simulink model "rect_v_RRC"  (R2014b)
settings: Solver=VariableStepDiscrete  StartTime=0.0  StopTime=5000/fs  RelTol=1e-3
PreLoadFcn:
  | %%%%%%%%%%%%%%%%%%%%%%%%%%%%%%%%%%%%%%%%%%%%%%%%%%%%%%%%%%%%%%%%%%%%%%%%%%%
  | % check to see if Simulink library folder is missing from the MATLAB path %
  | %%%%%%%%%%%%%%%%%%%%%%%%%%%%%%%%%%%%%%%%%%%%%%%%%%%%%%%%%%%%%%%%%%%%%%%%%%%
  | if isempty(strfind(path, 'rtlsdr_book_library'))
  | 
  |     % create error window
  |     fig_error = figure(...
  |         'Name', 'Error: RTL-SDR Book Library',...
  |         'Toolbar','none',...
  |         'MenuBar','none',...
  |         'NumberTitle','off',...
  |         'Resize','off',...
  |         'WindowStyle','modal');
  |     fig_error.Position(3) = 600;
  |     fig_error.Position(4) = 150;
  |     fig_axes = axes(...
  |         'Parent',fig_error,...
  |         'Position',[0,0,1,1],...
  |         'visible','off');
  |     % error message
  |     t_title = text(.05,.8,...
  |         'MISSING DIRECTORIES',...
  |         'FontSize',11.5);
  |     t_body = text(.075,.6,...
  |         [{'Simulink cannot find the  \it{<root>}\rm / \it{rtlsdr\_book\_library}\rm  folder in the \it{MATLAB Path}\rm.'},...
  |         {'Please set the MATLAB path following the instructions given in Exercise 2.4.'}],...
  |         'FontSize',10.5);
  |     % buttons
  |     btn_path = uicontrol(...
  |         'Parent',fig_error,...
  |         'String','Set Path Now',...
  |         'FontSize',10,...
  |         'Callback', 'pathtool; close(fig_error);',...
  |         'Position', [fig_error.Position(3)/2-210, 30, 200, 30]);
  |     btn_abort = uicontrol(...
  |         'Parent',fig_error,...
  |         'String','No thanks',...
  |         'FontSize',10,...
  |         'Callback', 'close(fig_error); abort=1;',...
  |         'Position', [fig_error.Position(3)/2+10, 30, 200, 30]);
  | 
  |     % pause to allow user to interact with error box
  |     uiwait(fig_error);
  | 
  |     % abort simulation
  |     try
  |         if abort==1
  |             set_param(gcs, 'SimulationCommand', 'stop');
  |         end
  |     end
  | 
  |     % if user has set path, allow diagram to be updated
  |     if ~exist('abort','var')
  |         % create error window
  |         fig_update = figure(...
  |             'Name', 'Update Diagram',...
  |             'Toolbar','none',...
  |             'MenuBar','none',...
  |             'NumberTitle','off',...
  |             'Resize','off');
  |         fig_update.Position(3) = 400;
  |         fig_update.Position(4) = 120;
  |         fig_axes = axes(...
  |             'Parent',fig_update,...
  |             'Position',[0,0,1,1],...
  |             'visible','off');
  |         % instruction message
  |         t_body = text(.075,.7,...
  |             'Once you have set the path, update the block diagram',...
  |             'FontSize',10.5);
  |         % button
  |         btn_update = uicontrol(...
  |             'Parent',fig_update,...
  |             'String','Update Block Diagram',...
  |             'FontSize',10,...
  |             'Callback', 'set_param(gcs,''SimulationCommand'',''update''); close(gcf)',...
  |             'Position', [fig_update.Position(3)/2-100, 30, 200, 30]);
  |     end
  | 
  |     % clear error components
  |     clear('fig_error','fig_update','fig_axes','t_title','t_body','btn_path','btn_abort','btn_update','abort');
  | 
  | end
  | %%%%%%%%%%%%%%%%%%%%%%%%%%%%%%%%%%%%%%%%%%%%%%%%%%%%%%%%%%%%%%%%%%%%%%%%%%%
  | 
  | 
  | MHz = 100;
  | fs = MHz * 1e6;
  | 
  | % parameters for filter design
  | OSR = 8;               % samples per symbol
  | Symbols = 10;        % symbol periods
  | Rolloff = 0.25;       % rolloff rate
  | 
  | % specify and design filter object
  | dRRC = fdesign.pulseshaping(OSR,'Square Root Raised Cosine','Nsym,Beta',Symbols,Rolloff);
  | hRRC = design(dRRC);
undefined symbols (not defined in the file): fdesignblkfcn, gcbh, startfcn_spectrum_analyzer, startfcn_time_scope
libraries: dspsigops x4, commrandsrc2 x1, rtlsdr_book_library x1, commdigbbndpm3 x1
CloseFcn:
  | closefcn_model;
Description:
  | Software, Simulation Examples and Design Exercises Licence Agreement
  | 
  | This license agreement refers to the simulation examples, design exercises and files,
  | and associated software MATLAB and Simulink resources that accompany the book:
  | 
  |      Title: Software Defined Radio using MATLAB & Simulink and the RTL-SDR
  |      Published by Strathclyde Academic Media, 2015
  |      Authored by Robert W. Stewart, Kenneth W. Barlee, Dale S.W. Atkinson,
  |      and Louise H. Crockett
  | 
  | and made available as a download from, www.desktopSDR.com or variously acquired
  | by other means such as via USB storage, cloud storage, disk or any other electronic
  | or optical or magnetic storage mechanism. These files and associated software may
  | be used subject to the terms of agreement of the conditions below:
  | 
  |     Copyright © 2015 Robert W. Stewart, Kenneth W. Barlee, Dale S.W. Atkinson,
  |     and Louise H. Crockett
  |     All rights reserved.
  | 
  | Redistribution and use in source and binary forms, with or without modification, are
  | permitted provided that the following conditions are met:
  | 
  |    1.  Redistributions of source code must retain the above copyright notice, this list of
  |         conditions and the following disclaimer.
  | 
  |    2.  Redistributions in binary form must reproduce the above copyright notice, this
  |         list of conditions and the following disclaimer in the documentation and/or other
  |         materials provided with the distribution.
  | 
  |    3.  Neither the name of the copyright holder nor the names of its contributors may
  |         be used to endorse or promote products derived from this software without
  |         specific prior written permission.
  | 
  |    4.  In all cases, the software is, and all modifications and derivatives of the
  |         software shall be, licensed to you solely for use in conjunction with The
  |         MathWorks, Inc. products and service offerings.
  | 
  | THIS SOFTWARE IS PROVIDED BY THE COPYRIGHT HOLDERS AND CONTRIBUTORS
  | "AS IS" AND ANY EXPRESS OR IMPLIED WARRANTIES, INCLUDING, BUT NOT LIMITED
  | TO, THE IMPLIED WARRANTIES OF MERCHANTABILITY AND FITNESS FOR A
  | PARTICULAR PURPOSE ARE DISCLAIMED. IN NO EVENT SHALL THE COPYRIGHT
  | HOLDER OR CONTRIBUTORS BE LIABLE FOR ANY DIRECT, INDIRECT, INCIDENTAL,
  | SPECIAL, EXEMPLARY, OR CONSEQUENTIAL DAMAGES (INCLUDING, BUT NOT
  | LIMITED TO, PROCUREMENT OF SUBSTITUTE GOODS OR SERVICES; LOSS OF USE,
  | DATA, OR PROFITS; OR BUSINESS INTERRUPTION) HOWEVER CAUSED AND ON ANY
  | THEORY OF LIABILITY, WHETHER IN CONTRACT, STRICT LIABILITY, OR TORT
  | (INCLUDING NEGLIGENCE OR OTHERWISE) ARISING IN ANY WAY OUT OF THE USE
  | OF THIS SOFTWARE, EVEN IF ADVISED OF THE POSSIBILITY OF SUCH DAMAGE.
  | 
  | 
  | Audio Tracks used in Simulations Examples and Design Exercises
  | 
  | The music and vocal files used within the Examples files and software within the book
  | were variously written, arranged, performed, recorded and produced by Garrey Rice,
  | Adam Struth, Jamie Struth, Iain Thistlethwaite and also Marshall Craigmyle who
  | collectively, and individually where appropriate, assert and retain all of their copyright,
  | performance and artistic rights. Permission to use and reproduce this music is
  | granted for all purposes associated with MATLAB and Simulink software and the
  | simulation examples and design exercises files that accompany this book. Requests to
  | use the music for any other purpose should be directed to: info@desktopSDR.com.
  | For information on music track names, full credits, and links to the musicians please
  | refer to www.desktopSDR.com/more/audio.
settings Model: Creator=desktopSDR Team  LastModifiedBy=desktopSDR Team
settings DataIOCC: LimitDataPoints=off  SaveOutput=off  SignalLogging=off  SaveTime=off
settings OptimizationCC: BlockReduction=off  ConditionallyExecuteInputs=off  InlineParams=on
settings DebuggingCC: AlgebraicLoopMsg=error  UnderspecifiedInitializationDetection=Classic  MergeDetectMultiDrivingBlocksExec=none
settings HardwareCC: ProdHWDeviceType=ASIC/FPGA->ASIC/FPGA  ProdEqTarget=off

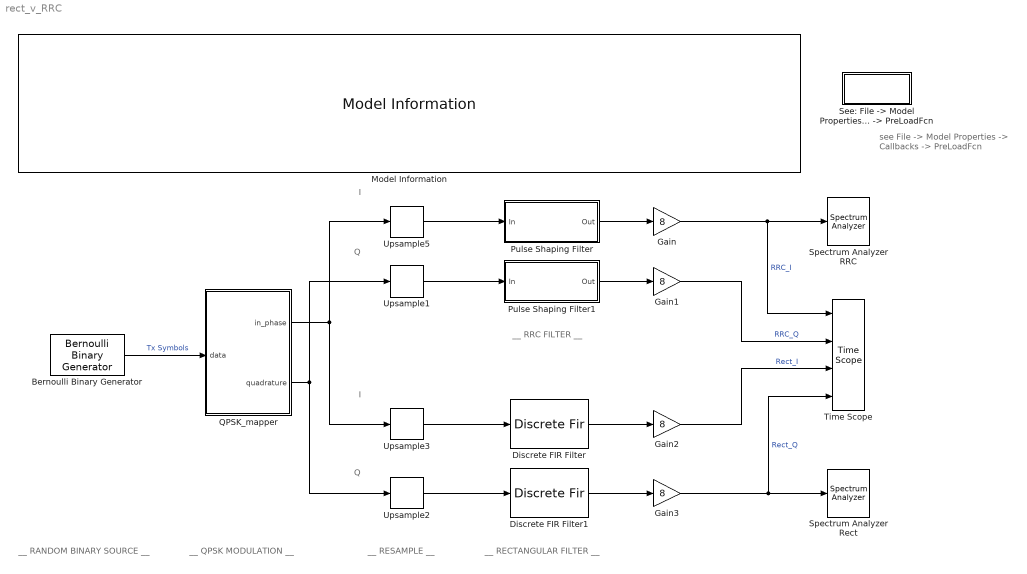
== system rect_v_RRC ==
  note: I
  note: see File -> Model Properties
      | -> Callbacks -> PreLoadFcn
  note: Q
  note: I
  note: Q
  note: __ RANDOM BINARY SOURCE __
  note: __ QPSK MODULATION __
  note: __ RECTANGULAR FILTER __
  note: __ RESAMPLE __
  note: __ RRC FILTER __
  Bernoulli Binary Generator : commrandsrc2/Bernoulli Binary Generator  P=0.5  seed=61  Ts=4/fs  frameBased=on  sampPerFrame=2  orient=off  outDataType=boolean
  Discrete FIR Filter : DiscreteFir  Coefficients=[1 1 1 1 1 1 1 1]  InputProcessing=Columns as channels (frame based)
  Discrete FIR Filter1 : DiscreteFir  Coefficients=[1 1 1 1 1 1 1 1]  InputProcessing=Columns as channels (frame based)
  Gain{,1..3} (4 alike) : Gain  Gain=8
  Model Information : rtlsdr_book_library/Additional Tools/Model Information/Model Information
  Pulse Shaping Filter : Subsystem  DialogController=fdesignblkfcn  InitFcn=fdesignblkfcn(gcbh, {'InitFcn'});  mask(Pulse Shaping Filter){}
      mask help: Design a Pulse Shaping Filter
      settings: CopyFcn=fdesignblkfcn(gcbh, {'CopyFcn'});
      mask Help: helpview(mapfilelocation('dsp'), 'dsppulseshapingfilter');
      mask Display: disp('Pulse Shaping');
  Pulse Shaping Filter1 : Subsystem  DialogController=fdesignblkfcn  InitFcn=fdesignblkfcn(gcbh, {'InitFcn'});  mask(Pulse Shaping Filter){}
      mask help: Design a Pulse Shaping Filter
      settings: CopyFcn=fdesignblkfcn(gcbh, {'CopyFcn'});
      mask Help: helpview(mapfilelocation('dsp'), 'dsppulseshapingfilter');
      mask Display: disp('Pulse Shaping');
  QPSK_mapper : Subsystem
  "See: File -> Model Properties -> Callbacks -> PreLoadFcn " : Subsystem
      mask Display:
      | MHz = evalin('base', 'MHz');
      | fprintf(['fs = ',num2str(MHz),' MHz']);
  Spectrum Analyzer RRC : SpectrumAnalyzer  StartFcn=startfcn_spectrum_analyzer;
  Spectrum Analyzer Rect : SpectrumAnalyzer  StartFcn=startfcn_spectrum_analyzer;
  Time Scope : TimeScope  StartFcn=startfcn_time_scope;  DefaultConfigurationName=spbscopes.TimeScopeBlockCfg  NumInputPorts=4
  Upsample{1..3,5} (4 alike) : dspsigops/Upsample  N=OSR  phase=0  InputProcessing=Columns as channels (frame based)  RateOptions=Allow multirate processing  ic=0  mode=Unused parameter value
  wires:
  Bernoulli Binary Generator/1 -> QPSK_mapper/1(data)  "Tx Symbols"
  Gain/1 -> Spectrum Analyzer RRC/1, Time Scope/1  "RRC_I"
  Gain1/1 -> Time Scope/2  "RRC_Q"
  Pulse Shaping Filter/1(Out) -> Gain/1
  Upsample5/1 -> Pulse Shaping Filter/1(In)
  Pulse Shaping Filter1/1(Out) -> Gain1/1
  Upsample1/1 -> Pulse Shaping Filter1/1(In)
  QPSK_mapper/2(quadrature) -> Upsample1/1, Upsample2/1
  Gain2/1 -> Time Scope/3  "Rect_I"
  Gain3/1 -> Spectrum Analyzer Rect/1, Time Scope/4  "Rect_Q"
  Discrete FIR Filter/1 -> Gain2/1
  QPSK_mapper/1(in_phase) -> Upsample5/1, Upsample3/1
  Upsample3/1 -> Discrete FIR Filter/1
  Discrete FIR Filter1/1 -> Gain3/1
  Upsample2/1 -> Discrete FIR Filter1/1

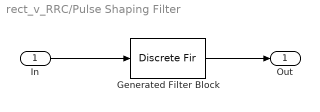
== system rect_v_RRC/Pulse Shaping Filter ==
  In : Inport
  Generated Filter Block : DiscreteFir  Tag=BlockMethodSubSystem  Coefficients=[-0.00093782949599698529 -0.0013563163010034674 -0.0014288038946264961 -0.0010885181024721721 -0.00036662864395568795 0.00060252468518526736 0.0016003936437970292 0.0023658487747616739 0.0026525823848649222 0.0022910053195207953 0.001241007000979448 -0.00037763636861196169 -0.0022870530417242589 -0.0040892242032672232 -0.0053366436064254614 -0.0056247462628233914 -0.0046891474799849227 -0.0024876020813169339 0.00075271731147288164 0.0045372796098467789 0.0081620180181291215 0.010822945010982432 0.011762888784769054 0.010431754588869383 0.0066314559621623017 0.00061639728402609157 -0.006874415523566337 -0.014667449373785968 -0.021287204230749861 -0.025156894374454848 -0.024839671278605167 -0.019283534116185753 -0.0080296444721248243 0.0086528817341815084 0.02973272866437043 0.053494676902035861 0.077724676313641453 0.099978396595261809 0.11789566509304776 0.12951468163808511 0.13353873577297384 0.12951468163808511 0.11789566509304776 0.099978396595261809 0.077724676313641453 0.053494676902035861 0.02973272866437043 0.0086528817341815084 -0.0080296444721248243 -0.019283534116185753 -0.024839671278605167 -0.025156894374454848 -0.021287204230749861 -0.014667449373785968 -0.006874415523566337 0.00061639728402609157 0.0066314559621623017 0.010431754588869383 0.011762888784769054 0.010822945010982432 0.0081620180181291215 0.0045372796098467789 0.00075271731147288164 -0.0024876020813169339 -0.0046891474799849227 -0.0056247462628233914 -0.0053366436064254614 -0.0040892242032672232 -0.0022870530417242589 -0.00037763636861196169 0.001241007000979448 0.0022910053195207953 0.0026525823848649222 0.0023658487747616739 0.0016003936437970292 0.00060252468518526736 -0.00036662864395568795 -0.0010885181024721721 -0.0014288038946264961 -0.0013563163010034674 -0.00093782949599698529]  InputProcessing=Columns as channels (frame based)
  Out : Outport
  wires:
  In/1 -> Generated Filter Block/1
  Generated Filter Block/1 -> Out/1

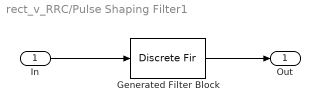
== system rect_v_RRC/Pulse Shaping Filter1 ==
  In : Inport
  Generated Filter Block : DiscreteFir  Tag=BlockMethodSubSystem  Coefficients=[-0.00093782949599698529 -0.0013563163010034674 -0.0014288038946264961 -0.0010885181024721721 -0.00036662864395568795 0.00060252468518526736 0.0016003936437970292 0.0023658487747616739 0.0026525823848649222 0.0022910053195207953 0.001241007000979448 -0.00037763636861196169 -0.0022870530417242589 -0.0040892242032672232 -0.0053366436064254614 -0.0056247462628233914 -0.0046891474799849227 -0.0024876020813169339 0.00075271731147288164 0.0045372796098467789 0.0081620180181291215 0.010822945010982432 0.011762888784769054 0.010431754588869383 0.0066314559621623017 0.00061639728402609157 -0.006874415523566337 -0.014667449373785968 -0.021287204230749861 -0.025156894374454848 -0.024839671278605167 -0.019283534116185753 -0.0080296444721248243 0.0086528817341815084 0.02973272866437043 0.053494676902035861 0.077724676313641453 0.099978396595261809 0.11789566509304776 0.12951468163808511 0.13353873577297384 0.12951468163808511 0.11789566509304776 0.099978396595261809 0.077724676313641453 0.053494676902035861 0.02973272866437043 0.0086528817341815084 -0.0080296444721248243 -0.019283534116185753 -0.024839671278605167 -0.025156894374454848 -0.021287204230749861 -0.014667449373785968 -0.006874415523566337 0.00061639728402609157 0.0066314559621623017 0.010431754588869383 0.011762888784769054 0.010822945010982432 0.0081620180181291215 0.0045372796098467789 0.00075271731147288164 -0.0024876020813169339 -0.0046891474799849227 -0.0056247462628233914 -0.0053366436064254614 -0.0040892242032672232 -0.0022870530417242589 -0.00037763636861196169 0.001241007000979448 0.0022910053195207953 0.0026525823848649222 0.0023658487747616739 0.0016003936437970292 0.00060252468518526736 -0.00036662864395568795 -0.0010885181024721721 -0.0014288038946264961 -0.0013563163010034674 -0.00093782949599698529]  InputProcessing=Columns as channels (frame based)
  Out : Outport
  wires:
  Generated Filter Block/1 -> Out/1
  In/1 -> Generated Filter Block/1

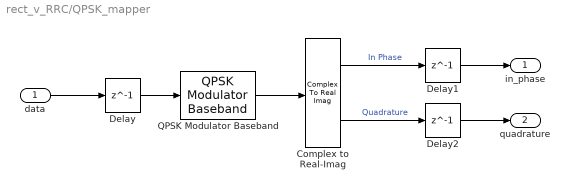
== system rect_v_RRC/QPSK_mapper ==
  data : Inport
  Complex to Real-Imag : ComplexToRealImag
  Delay : Delay  DelayLength=1  InputProcessing=Columns as channels (frame based)
  Delay1 : Delay  DelayLength=1  InputProcessing=Columns as channels (frame based)
  Delay2 : Delay  DelayLength=1  InputProcessing=Columns as channels (frame based)
  QPSK Modulator Baseband : commdigbbndpm3/QPSK Modulator Baseband  InType=Bit  Enc=Gray  Ph=pi/4  outDtype=double  outWordLen=16  outUDDataType=sfix(16)  outFracLenMode=User-defined  outFracLen=15
  in_phase : Outport
  quadrature : Outport  Port=2
  wires:
  data/1 -> Delay/1
  QPSK Modulator Baseband/1 -> Complex to Real-Imag/1
  Complex to Real-Imag/2 -> Delay2/1  "Quadrature"
  Complex to Real-Imag/1 -> Delay1/1  "In Phase"
  Delay/1 -> QPSK Modulator Baseband/1
  Delay1/1 -> in_phase/1
  Delay2/1 -> quadrature/1

== system rect_v_RRC/See: File -> Model Properties -> Callbacks -> PreLoadFcn  ==
